simulink model "Linear_Moving_Setpoint_SS_w_FF"  (R2021b)
settings: Solver=VariableStepAuto  StartTime=tspan(1)  StopTime=tspan(2)  RelTol=1e-9
undefined symbols (not defined in the file): K1, K2, r_sim
settings Model: Creator=domin  LastModifiedBy=domin
settings SolverCC: AlgebraicLoopSolver=TrustRegion
settings DebuggingCC: AlgebraicLoopMsg=none  SFMachineParentedDataDiag=warning

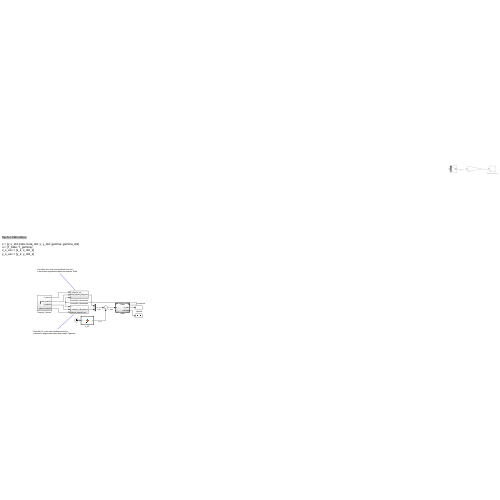
[thumbnail: Simulink's stored preview of the top-level diagram]
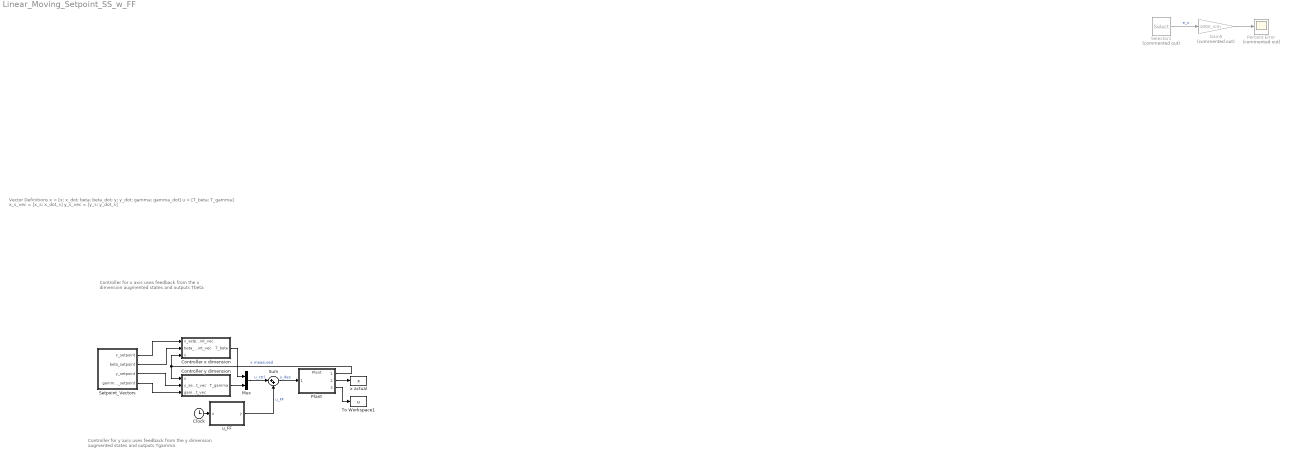
== system Linear_Moving_Setpoint_SS_w_FF ==
  note: Controller for y axis uses feedback from the
      | y dimension augmented states and outputs Tgamma
  note: Vector Definitions
      |
      | x = [x; x_dot; beta; beta_dot; y; y_dot; gamma; gamma_dot]
      | u = [T_beta; T_gamma]
      | x_s_vec = [x_s; x_dot_s]
      | y_s_vec = [y_s; y_dot_s]
  note: Controller for x axis uses feedback from the
      | x dimension augmented states and outputs Tbeta
  Clock : Clock
  Controller x dimension : Subsystem
  Controller y dimension : Subsystem
  Gain5 : Gain  Commented=on  Gain=100/r_sim
  Mux : Mux  Inputs=2
  Percent Error : Scope  Commented=on
  Plant : ModelReference  ModelNameDialog=Plant  SimulationMode=Normal  ModelReferenceVersion=1.56
  Selector1 : Selector  Commented=on  InputPortWidth=5  IndexOptions=Index vector (dialog)  Indices=[1]  OutputSizes=1
  Setpoint_Vectors : Subsystem
  Sum : Sum  Inputs=|++
  To Workspace1 : ToWorkspace  VariableName=u  SampleTime=-1
  u_FF : MATLAB Function  TreatAsAtomicUnit=on
  x actual : ToWorkspace  VariableName=x  SampleTime=-1
  wires:
  Gain5/1 -> Percent Error/1
  Selector1/1 -> Gain5/1  "e_x"
  Controller x dimension/1(T_beta) -> Mux/1
  Controller y dimension/1(T_gamma) -> Mux/2
  Mux/1 -> Sum/1  "u_ctrl"
  Plant/1 -> Controller x dimension/3(x), Controller y dimension/1(x)  "x measured"
  Plant/3 -> To Workspace1/1
  Plant/2 -> x actual/1
  Setpoint_Vectors/1(x_setpoint) -> Controller x dimension/1(x_setpoint_vec)
  Setpoint_Vectors/3(y_setpoint) -> Controller y dimension/2(y_setpoint_vec)
  Setpoint_Vectors/2(beta_setpoint) -> Controller x dimension/2(beta_setpoint_vec)
  Setpoint_Vectors/4(gamma_setpoint) -> Controller y dimension/3(gamma_setpoint_vec)
  Clock/1 -> u_FF/1(u)
  Sum/1 -> Plant/1  "u_des"
  u_FF/1(y) -> Sum/2  "u_FF"

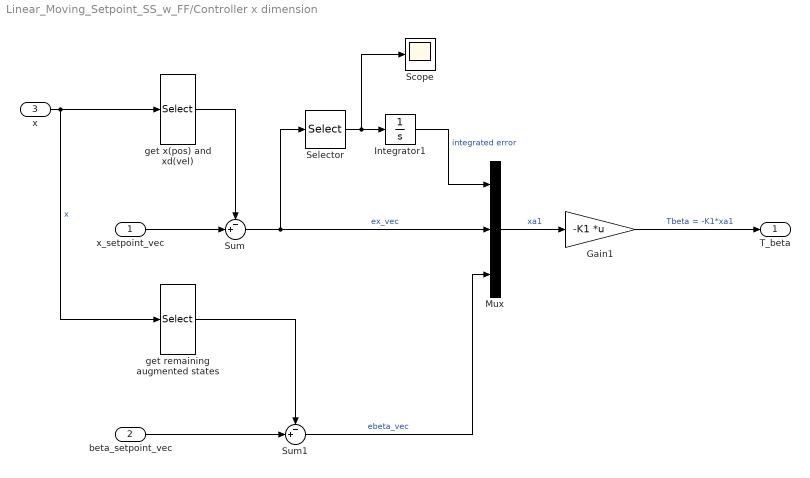
== system Linear_Moving_Setpoint_SS_w_FF/Controller x dimension ==
  x_setpoint_vec : Inport
  beta_setpoint_vec : Inport  Port=2
  x : Inport  Port=3
  Gain1 : Gain  Gain=-K1  Multiplication=Matrix(K*u)
  Integrator1 : Integrator
  Mux : Mux  Inputs=3
  Scope : Scope
  Selector : Selector  InputPortWidth=2  IndexOptions=Index vector (dialog)  Indices=[1 ]  OutputSizes=1
  Sum : Sum  Inputs=-+|
  Sum1 : Sum  Inputs=-+|
  get remaining augmented states : Selector  InputPortWidth=8  IndexOptions=Index vector (dialog)  Indices=[3,4]  OutputSizes=1
  get x(pos) and xd(vel) : Selector  InputPortWidth=8  IndexOptions=Index vector (dialog)  Indices=[1 2]  OutputSizes=1
  T_beta : Outport
  wires:
  get remaining augmented states/1 -> Sum1/1
  Gain1/1 -> T_beta/1  "Tbeta = -K1*xa1"
  get x(pos) and xd(vel)/1 -> Sum/1
  Mux/1 -> Gain1/1  "xa1"
  Sum/1 -> Selector/1, Mux/2  "ex_vec"
  x_setpoint_vec/1 -> Sum/2
  x/1 -> get x(pos) and xd(vel)/1, get remaining augmented states/1  "x"
  Selector/1 -> Scope/1, Integrator1/1
  Integrator1/1 -> Mux/1  "integrated error"
  beta_setpoint_vec/1 -> Sum1/2
  Sum1/1 -> Mux/3  "ebeta_vec"

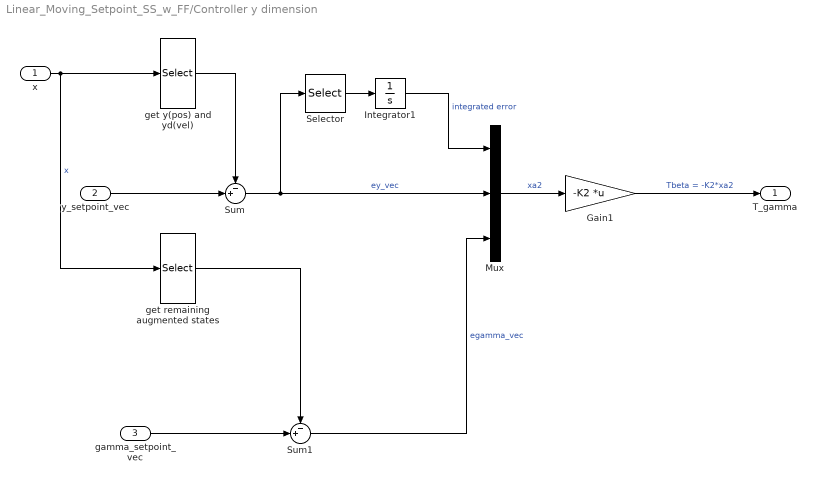
== system Linear_Moving_Setpoint_SS_w_FF/Controller y dimension ==
  x : Inport
  y_setpoint_vec : Inport  Port=2
  gamma_setpoint_vec : Inport  Port=3
  Gain1 : Gain  Gain=-K2  Multiplication=Matrix(K*u)
  Integrator1 : Integrator
  Mux : Mux  Inputs=3
  Selector : Selector  InputPortWidth=2  IndexOptions=Index vector (dialog)  Indices=[1 ]  OutputSizes=1
  Sum : Sum  Inputs=-+|
  Sum1 : Sum  Inputs=-+|
  get remaining augmented states : Selector  InputPortWidth=8  IndexOptions=Index vector (dialog)  Indices=[7,8]  OutputSizes=1
  get y(pos) and yd(vel) : Selector  InputPortWidth=8  IndexOptions=Index vector (dialog)  Indices=[5 6]  OutputSizes=1
  T_gamma : Outport
  wires:
  Integrator1/1 -> Mux/1  "integrated error"
  x/1 -> get y(pos) and yd(vel)/1, get remaining augmented states/1  "x"
  Gain1/1 -> T_gamma/1  "Tbeta = -K2*xa2"
  get y(pos) and yd(vel)/1 -> Sum/1
  Mux/1 -> Gain1/1  "xa2"
  Selector/1 -> Integrator1/1
  Sum/1 -> Selector/1, Mux/2  "ey_vec"
  y_setpoint_vec/1 -> Sum/2
  gamma_setpoint_vec/1 -> Sum1/2
  Sum1/1 -> Mux/3  "egamma_vec"
  get remaining augmented states/1 -> Sum1/1

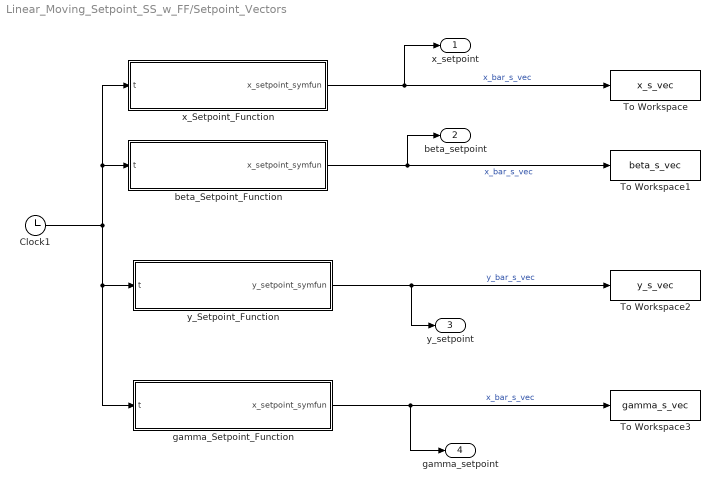
== system Linear_Moving_Setpoint_SS_w_FF/Setpoint_Vectors ==
  Clock1 : Clock
  To Workspace : ToWorkspace  VariableName=x_s_vec  SampleTime=-1
  To Workspace1 : ToWorkspace  VariableName=beta_s_vec  SampleTime=-1
  To Workspace2 : ToWorkspace  VariableName=y_s_vec  SampleTime=-1
  To Workspace3 : ToWorkspace  VariableName=gamma_s_vec  SampleTime=-1
  beta_Setpoint_Function : MATLAB Function  TreatAsAtomicUnit=on
  gamma_Setpoint_Function : MATLAB Function  TreatAsAtomicUnit=on
  x_Setpoint_Function : MATLAB Function  TreatAsAtomicUnit=on
  y_Setpoint_Function : MATLAB Function  TreatAsAtomicUnit=on
  x_setpoint : Outport
  beta_setpoint : Outport  Port=2
  y_setpoint : Outport  Port=3
  gamma_setpoint : Outport  Port=4
  wires:
  y_Setpoint_Function/1(y_setpoint_symfun) -> y_setpoint/1, To Workspace2/1  "y_bar_s_vec"
  Clock1/1 -> x_Setpoint_Function/1(t), beta_Setpoint_Function/1(t), gamma_Setpoint_Function/1(t), y_Setpoint_Function/1(t)
  x_Setpoint_Function/1(x_setpoint_symfun) -> x_setpoint/1, To Workspace/1  "x_bar_s_vec"
  beta_Setpoint_Function/1(x_setpoint_symfun) -> To Workspace1/1, beta_setpoint/1  "x_bar_s_vec"
  gamma_Setpoint_Function/1(x_setpoint_symfun) -> gamma_setpoint/1, To Workspace3/1  "x_bar_s_vec"

== matlab function Linear_Moving_Setpoint_SS_w_FF/Setpoint_Vectors/x_Setpoint_Function ==
  data: t input; x_setpoint_symfun output
function x_setpoint_symfun = x_setpoint(t)
%#codegen

%    This function was generated by the Symbolic Math Toolbox version 9.0.
%    18-Feb-2022 15:42:07

t2 = t./2.0;
t3 = (t.*pi)./3.0;
t4 = t.*pi.*(2.0./3.0);
t5 = -t2;
t7 = cos(t3);
t8 = cos(t4);
t6 = exp(t5);
t9 = t6-1.0;
x_setpoint_symfun = [t7.*t8.*t9.*(-3.0./1.0e+1);t6.*t7.*t8.*(3.0./2.0e+1)+(t7.*t9.*pi.*sin(t4))./5.0+(t8.*t9.*pi.*sin(t3))./1.0e+1];

== matlab function Linear_Moving_Setpoint_SS_w_FF/Setpoint_Vectors/y_Setpoint_Function ==
  data: t input; y_setpoint_symfun output
function y_setpoint_symfun = y_setpoint(t)
%#codegen

%    This function was generated by the Symbolic Math Toolbox version 9.0.
%    18-Feb-2022 15:42:07

t2 = t./2.0;
t3 = (t.*pi)./3.0;
t4 = t.*pi.*(2.0./3.0);
t5 = -t2;
t7 = cos(t4);
t8 = sin(t3);
t6 = exp(t5);
t9 = t6-1.0;
y_setpoint_symfun = [t7.*t8.*t9.*(-3.0./1.0e+1);t6.*t7.*t8.*(3.0./2.0e+1)-(t7.*t9.*pi.*cos(t3))./1.0e+1+(t8.*t9.*pi.*sin(t4))./5.0];

== matlab function Linear_Moving_Setpoint_SS_w_FF/Setpoint_Vectors/gamma_Setpoint_Function ==
  data: t input; x_setpoint_symfun output
function x_setpoint_symfun = x_setpoint(t)
%#codegen

%    This function was generated by the Symbolic Math Toolbox version 9.0.
%    18-Feb-2022 15:42:07

t2 = t./2.0;
t3 = (t.*pi)./3.0;
t4 = t.*pi.*(2.0./3.0);
t5 = -t2;
t7 = cos(t3);
t8 = cos(t4);
t6 = exp(t5);
t9 = t6-1.0;
x_setpoint_symfun = [t7.*t8.*t9.*(-3.0./1.0e+1);t6.*t7.*t8.*(3.0./2.0e+1)+(t7.*t9.*pi.*sin(t4))./5.0+(t8.*t9.*pi.*sin(t3))./1.0e+1];

== matlab function Linear_Moving_Setpoint_SS_w_FF/u_FF ==
  data: u input; y output
function y = fcn(u)

y = u;

== matlab function Linear_Moving_Setpoint_SS_w_FF/Setpoint_Vectors/beta_Setpoint_Function ==
  data: t input; x_setpoint_symfun output
function x_setpoint_symfun = x_setpoint(t)
%#codegen

%    This function was generated by the Symbolic Math Toolbox version 9.0.
%    18-Feb-2022 15:42:07

t2 = t./2.0;
t3 = (t.*pi)./3.0;
t4 = t.*pi.*(2.0./3.0);
t5 = -t2;
t7 = cos(t3);
t8 = cos(t4);
t6 = exp(t5);
t9 = t6-1.0;
x_setpoint_symfun = [t7.*t8.*t9.*(-3.0./1.0e+1);t6.*t7.*t8.*(3.0./2.0e+1)+(t7.*t9.*pi.*sin(t4))./5.0+(t8.*t9.*pi.*sin(t3))./1.0e+1];
